simulink model "Microgrid_24h_Simulation"  (Simulink 9.3)
settings: Solver=ode45  StartTime=0.0  StopTime=1  RelTol=1e-3  EnableMultiTasking=on
undefined symbols (not defined in the file or in its folder): Acid, Lead
libraries: powerlib x60, powerlib_extras x56, simulink x3, powerlib_meascontrol x2, electricdrivelib x1
(part 3 of 3)

== system Microgrid_24h_Simulation/Subsystem/Subsystem11/Load Power Calculation2/Subsystem2 ==
  Pload : Inport
  LPF vq7 : powerlib_extras/Discrete  Control Blocks/Discrete 1st-Order Filter  FilterType=Lowpass  Tc=10e-3  Ts=5e-6  Initialize=off  Vac_Init=[0.8 -25 60]  Vdc_Init=0  PlotResponse=off  param1=[1 100 0.1]
      settings: SourceProductName=Simscape Electrical  SourceProductBaseCode=PS
  To Workspace1 : ToWorkspace  VariableName=Pacload2  SampleTime=-1
  To Workspace2 : ToWorkspace  VariableName=Pacload_2  SampleTime=-1
  Zero-Order Hold : ZeroOrderHold  SampleTime=5e-6
  tag scope: Pacload2=global
  wires:
  Pload/1 -> Zero-Order Hold/1
  Zero-Order Hold/1 -> [Pacload2], To Workspace2/1, LPF vq7/1
  LPF vq7/1 -> To Workspace1/1

== system Microgrid_24h_Simulation/Subsystem/Inverter Control  Measurements3/PLL/abc  - d/q/abc  - alfa/beta ==
  abc : Inport
  Mux : Mux  Inputs=2
  d_s : Fcn  Expr=(-1/sqrt(3)*u[2])+(1/sqrt(3)*u[3])
  q_s : Fcn  Expr=(2/3)*u[1]-(1/3)*u[2]-(1/3)*u[3]
  alfa/beta : Outport
  wires:
  abc/1 -> q_s/1, d_s/1
  d_s/1 -> Mux/1
  q_s/1 -> Mux/2
  Mux/1 -> alfa/beta/1

== system Microgrid_24h_Simulation/Subsystem/Inverter Control  Measurements3/PLL/abc  - d/q/alfa/beta - dq ==
  alfa/beta : Inport
  tita : Inport  Port=2
  Mux : Mux  Inputs=2
  Mux1 : Mux  Inputs=2
  d : Fcn  Expr=u[2]*sin(u[3]) + u[1]*cos(u[3])
  q : Fcn  Expr=-u[1]*sin(u[3]) + u[2]*cos(u[3])
  d/q : Outport
  wires:
  d/1 -> Mux/1
  q/1 -> Mux/2
  Mux/1 -> d/q/1
  alfa/beta/1 -> Mux1/1
  tita/1 -> Mux1/2
  Mux1/1 -> d/1, q/1

== matlab function PV Array/PV ==
  data: Vpv input double; Ipv output double; Irr input double; TaC input double
function Ipv = Photovoltaic(Vpv,Irr,TaC)

%% REFERENCE PAPER:
% Francisco M. González-Longatt, "Model of Photovoltaic Module inMatlabTM",
% II CIBELEC 2005.

%% Solar panel: Suntech STP-280S
% photovoltaic.m function calculates solar array current with a 
% given voltage, irradiance and temperature
% Ipv = photovoltaic array current (function output)
% Vpv = photovoltaic array voltage
% Irr = irradiance (1 Irr = 1000 W/m^2)
% TaC = temperature (in celsius degrees)

%% Constants

k = 1.38e-23;        % Boltzman’s const
q = 1.60e-19;        % charge on an electron
Np = 10;             % Number of solar panels
n = 2;               % Diode quality factor (=2 for crystaline, <2 for amorphous)
Vg = 1.12;           % Band gap voltage, 1.12V for xtal Si, 1.75 for amorphous Si
Ns = 72*Np;          % Number of cells conected in series (96 cells each panel) 96
T1 = 273 + 25;       % 25C degrees in Kelvin's
Voc_T1 = 44.8*Np/Ns; % Open circuit voltage per cell at T1 temperature 64.2
Isc_T1 = 8.33;       % Short circuit current at temperature T1 5.96

T2 = 273 + 75;
Voc_T2 = Voc_T1*(-0.34/100*(T2-T1)) /Ns; % Open circuit voltage per cell at temperature T2
Isc_T2 = Isc_T1*(0.05/100*(T2-T1));      % Short circuit current per cell at temperature T2

TaK = 273 + TaC; % Photovoltaic array working temperature
TrK = 273 + 25;  % Reference temperature

%% Calculation of the photocurrent Iph
K0 = (Isc_T2 - Isc_T1)/(T2-T1);          % K0 constant is determined from Isc vs T (ECUATION 4)
Iph_T1 = Isc_T1 * Irr;                   % (ECUATION 3)
Iph = Iph_T1 + K0*(TaK-T1);              % Photocurrent (ECUATION 2)

%% Calculation of saturation current of the diode I0
I0_T1 = Isc_T1/(exp(q*Voc_T1/(n*k*T1))-1);                       % (ECUATION 6)
I0 = I0_T1*(TaK/T1).^(3/n).*exp(-q*Vg/(n*k).*((1./TaK)-(1/T1))); % Diode sat. current

%% Calculation of the series resistance Rs, represents the resistance inside
%  its cell in the connection between cells
Xv = I0_T1*q/(n*k*T1)*exp(q*Voc_T1/(n*k*T1)); % (ECUATION 8)
dVdI_Voc = -1.15/Ns /2;                       % dV/dI at Vco per cell, from manufacturers graph
Rs = -dVdI_Voc - 1/Xv;                        % Resistance per cell (ECUATION 7)

%% Calculation of the PV array current, Ipv
Vt_Ta = n*k*TaK/q;                            % = nkT/q
Vc = Vpv/Ns;
Ipv = zeros(size(Vc));
% Ipv = Iph - I0.*( exp((Vc+Ipv.*Rs)./Vt_Ta) -1) (ECUATION 1);
% Solve for Ipv: f(Ipv) = Iph - Ipv - I0.*( exp((Vc+Ia.*Rs)./Vt_Ta) -1) = 0;
% Newton-Raphson method: Ipv2 = Ipv1 - f(Ipv1)/f’(Ipv1)
for j=1:5;
  Ipv = Ipv - ...
  (Iph - Ipv - I0.*( exp((Vc+Ipv.*Rs)./Vt_Ta) -1))...
  ./ (-1 - (I0.*( exp((Vc+Ipv.*Rs)./Vt_Ta) -1)).*Rs./Vt_Ta);
end

== matlab function Boost/Incremental Conductance MPPT/MPPT IC ==
  data: delta output double; Ipv input double; Iprevious input double; Vref output double; Vpv input double; Vprevious input double; Vref_previous input double; Ipv_prev_out output double; Vpv_prev_out output double
function [delta,Vref,Ipv_prev_out,Vpv_prev_out] = IncCond(Ipv,Iprevious,Vpv,Vprevious,Vref_previous)

% REFERENCE PAPERS:
% Trishan Esram, Patrick L. Chapman, "Comparison of Photovoltaic Array
% Maximum Power Tracking Techniques", IEEE Transactions on Energy
% COnversion, vol. 22, issue 2, June 2007.
%
% M. Lokanadham, K. Vijaya Bhaskar, "Incremental Conductance Based Maximum
% Power Point Tracking (MPPT) for Photovoltaic System" International
% Journal of Engineering Research and Applications (IJERA), vol. 2, issue
% 2, March-April 2012.


% The followoing code is an algorithm for a Maximum Power Point Tracking
% (MPPT) technique Incremental COnductance

Vbus = 600;

dI=Ipv-Iprevious;
dV=Vpv-Vprevious;

if (dV==0)
    if (dI==0)
        Vref=Vref_previous;
    else
        if (Ipv>0)
            Vref= Vpv+dV;
        else
            Vref= Vpv-dV;
        end
    end
else
    if ((dI/dV)==(-Ipv/Vpv))
        Vref=Vref_previous;
    else
        if ((dI/dV)>(-Ipv/Vpv))
            Vref= Vpv+dV;
        else
            Vref= Vpv-dV;
        end
    end
end
Ipv_prev_out=Ipv;
Vpv_prev_out=Vpv;

delta=1-Vref/Vbus;

end
